simulink model "ClosedLoopStepResp_FBD"  (Simulink 7.4)
settings: Solver=ode45  StartTime=0.0  StopTime=r0_L*Ts  RelTol=1e-3
values from neighbouring files (symbols this model uses):
  alpha = 10    [simModel.m]
  den = [40 1]    [simModel.m]
  Kc = 0.7    [simModel.m]
  n_den = 1    [simModel.m]
  n_num = 1    [simModel.m]
  num = 1.25    [simModel.m]
  nvar = 1*0.001    (= 0.001)    [simModel.m]
  Td = 0    [simModel.m]
  theta = 2    [simModel.m]
  Ti = 20    [simModel.m]
  Ts = 1    [simModel.m]
settings Model: Creator=Jiandong  LastModifiedBy=user

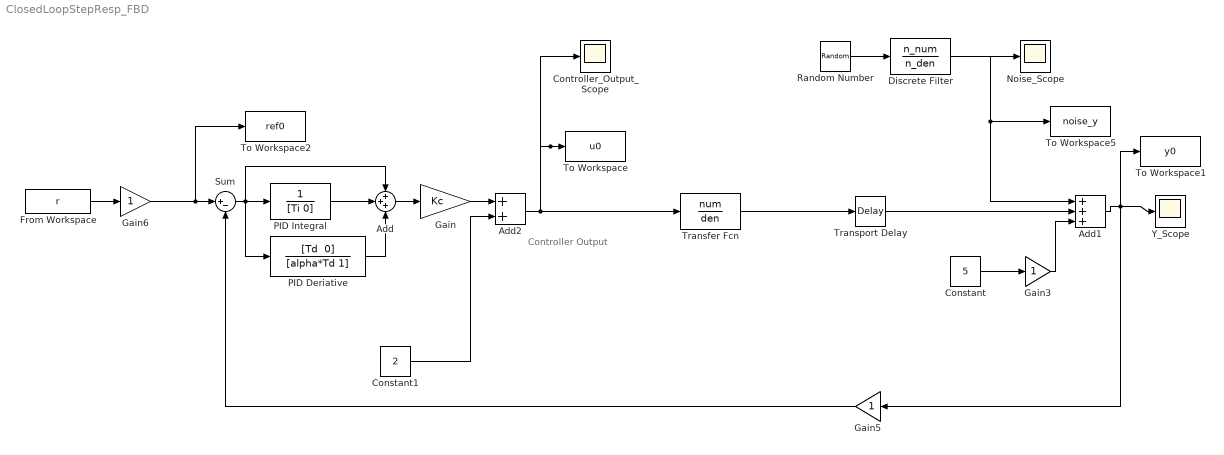
== system ClosedLoopStepResp_FBD ==
  note: Controller
      | Output
  Add : Sum  Inputs=+++  OutDataType=fixdt(1, 16)  OutScaling=2^-10
  Add1 : Sum  Inputs=+++  OutDataType=fixdt(1, 16)  OutScaling=2^-10
  Add2 : Sum  OutDataType=fixdt(1, 16)  OutScaling=2^-10
  Constant : Constant  Value=5  OutDataType=fixdt(1, 16)  OutScaling=2^0
  Constant1 : Constant  Value=2  OutDataType=fixdt(1, 16)  OutScaling=2^0
  Controller_Output_Scope : Scope
      settings: MaxDataPoints=50000
  Discrete Filter : DiscreteFilter  Numerator=n_num  Denominator=n_den  SampleTime=Ts
  From Workspace : FromWorkspace  VariableName=r  SampleTime=Ts
  Gain : Gain  Gain=Kc  ParameterDataType=fixdt(1, 16)  ParameterScaling=2^0  OutDataType=fixdt(1, 16)  OutScaling=2^0
  Gain3 : Gain  ParameterDataType=fixdt(1, 16)  ParameterScaling=2^0  OutDataType=fixdt(1, 16)  OutScaling=2^0
  Gain5 : Gain  ParameterDataType=fixdt(1, 16)  ParameterScaling=2^0  OutDataType=fixdt(1, 16)  OutScaling=2^0
  Gain6 : Gain  ParameterDataType=fixdt(1, 16)  ParameterScaling=2^0  OutDataType=fixdt(1, 16)  OutScaling=2^0
  Noise_Scope : Scope
      settings: SaveName=ScopeData2
  PID Deriative : TransferFcn  Numerator="[Td  0]"  Denominator=[alpha*Td 1]
  PID Integral : TransferFcn  Denominator=[Ti 0]
  Random Number : RandomNumber  Variance=nvar  SampleTime=Ts
  Sum : Sum  Inputs=|+-  OutDataType=fixdt(1, 16)  OutScaling=2^0
  To Workspace : ToWorkspace  VariableName=u0  SampleTime=Ts  SaveFormat=Structure With Time
  To Workspace1 : ToWorkspace  VariableName=y0  SampleTime=Ts  SaveFormat=Structure With Time
  To Workspace2 : ToWorkspace  VariableName=ref0  SampleTime=Ts  SaveFormat=Structure With Time
  To Workspace5 : ToWorkspace  VariableName=noise_y  SampleTime=Ts  SaveFormat=Structure With Time
  Transfer Fcn : TransferFcn  Numerator=num  Denominator=den
  Transport Delay : TransportDelay  DelayTime=theta
  Y_Scope : Scope
      settings: YMin=9.3  YMax=10.7  MaxDataPoints=50000
  wires:
  Add/1 -> Gain/1
  Sum/1 -> PID Integral/1, PID Deriative/1, Add/1
  PID Deriative/1 -> Add/3
  PID Integral/1 -> Add/2
  Discrete Filter/1 -> Noise_Scope/1, Add1/1, To Workspace5/1
  Add1/1 -> Y_Scope/1, To Workspace1/1, Gain5/1
  Constant/1 -> Gain3/1
  Add2/1 -> To Workspace/1, Controller_Output_Scope/1, Transfer Fcn/1
  Constant1/1 -> Add2/2
  Gain/1 -> Add2/1
  From Workspace/1 -> Gain6/1
  Gain6/1 -> Sum/1, To Workspace2/1
  Random Number/1 -> Discrete Filter/1
  Gain5/1 -> Sum/2
  Transfer Fcn/1 -> Transport Delay/1
  Transport Delay/1 -> Add1/2
  Gain3/1 -> Add1/3
